simulink model "saturazione2"  (R2017a)
settings: Solver=VariableStepAuto  StartTime=0.0  StopTime=15  RelTol=1e-3
settings Model: Creator=Enrico Donato  LastModifiedBy=Enrico Donato

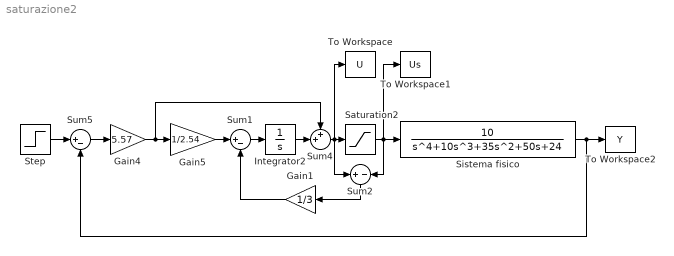
== system saturazione2 ==
  Gain1 : Gain  Gain=1/3
  Gain4 : Gain  Gain=5.57
  Gain5 : Gain  Gain=1/2.54
  Integrator2 : Integrator
  Saturation2 : Saturate  UpperLimit=3  LowerLimit=-3
  Sistema fisico : TransferFcn  Numerator=[10]  Denominator=[1 10 35 50 24]
  Step : Step  Time=0  SampleTime=0
  Sum1 : Sum  Inputs=|+-
  Sum2 : Sum  Inputs=+-
  Sum4 : Sum  Inputs=++|
  Sum5 : Sum  Inputs=|+-
  To Workspace : ToWorkspace  VariableName=U  SampleTime=-1
  To Workspace1 : ToWorkspace  VariableName=Us  SampleTime=-1
  To Workspace2 : ToWorkspace  VariableName=Y  SampleTime=-1
  wires:
  Saturation2/1 -> To Workspace1/1, Sum2/2, Sistema fisico/1
  Sistema fisico/1 -> To Workspace2/1, Sum5/2
  Sum5/1 -> Gain4/1
  Integrator2/1 -> Sum4/2
  Sum4/1 -> To Workspace/1, Sum2/1, Saturation2/1
  Step/1 -> Sum5/1
  Gain4/1 -> Sum4/1, Gain5/1
  Gain5/1 -> Sum1/1
  Sum1/1 -> Integrator2/1
  Sum2/1 -> Gain1/1
  Gain1/1 -> Sum1/2
